simulink subsystem "block_triad"  (R2019b)
settings: Solver=VariableStepAuto  StartTime=0.0  StopTime=10.0  RelTol=1e-3
libraries: blocklib x1
settings Model: Creator=imanol  LastModifiedBy=imanol

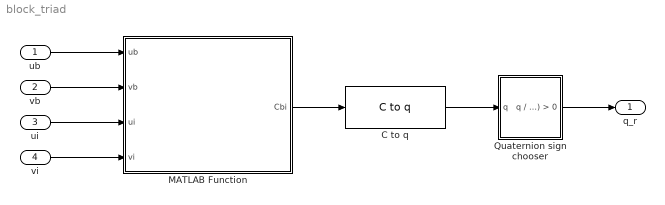
== system block_triad ==
  ub : Inport
  vb : Inport  Port=2
  ui : Inport  Port=3
  vi : Inport  Port=4
  C to q : blocklib/C to q  SystemSampleTime=-1  Latency=0  AutoFrameSizeCalculation=off
      settings: SourceProductName=Custom Library
  MATLAB Function : MATLAB Function  TreatAsAtomicUnit=on
  Quaternion sign chooser : Subsystem
  q_r : Outport
  wires:
  vb/1 -> MATLAB Function/2(vb)
  ub/1 -> MATLAB Function/1(ub)
  ui/1 -> MATLAB Function/3(ui)
  vi/1 -> MATLAB Function/4(vi)
  MATLAB Function/1(Cbi) -> C to q/1
  C to q/1 -> Quaternion sign chooser/1(q)
  Quaternion sign chooser/1(q / q(4) > 0) -> q_r/1

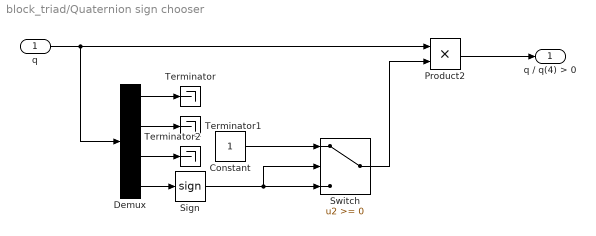
== system block_triad/Quaternion sign chooser ==
  q : Inport
  Constant : Constant
  Demux : Demux
  Product2 : Product
  Sign : Signum
  Switch : Switch
  Terminator : Terminator
  Terminator1 : Terminator
  Terminator2 : Terminator
  q / q(4) > 0 : Outport
  wires:
  Demux/3 -> Terminator2/1
  Switch/1 -> Product2/2
  Constant/1 -> Switch/1
  Demux/2 -> Terminator1/1
  Sign/1 -> Switch/3, Switch/2
  Demux/4 -> Sign/1
  Product2/1 -> q / q(4) > 0/1
  q/1 -> Product2/1, Demux/1
  Demux/1 -> Terminator/1

== matlab function block_triad/MATLAB Function ==
  data: ub input; Cbi output; vb input; ui input; vi input
function Cbi = TRIAD_MATRIX(ub, vb, ui, vi)

ub_norm = ub/norm(ub);
vb_norm = vb/norm(vb);

t1b = ub_norm;
t2b = cross(ub_norm,vb_norm);
t2b = t2b / norm(t2b);
t3b = cross(t1b,t2b);


ui_norm = ui/norm(ui);
vi_norm = vi/norm(vi);

t1i = ui_norm;
t2i = cross(ui_norm,vi_norm);
t2i = t2i / norm(t2i);
t3i = cross(t1i,t2i);

Cbi = [t1b t2b t3b]*[t1i t2i t3i]';

% phi = acos(0.5*(Cbi(1,1) + Cbi(2,2) + Cbi(3,3) -1));
% e = 1/(2*sin(phi))*[Cbi(2,3)-Cbi(3,2); Cbi(3,1) - Cbi(1,3); Cbi(1,2) - Cbi(2,1)];
% 
% q = [e*sin(phi/2);cos(phi/2)];

end
